simulink model "fullStateFeedback"  (R2019b)
settings: Solver=VariableStepAuto  StartTime=0.0  StopTime=3  RelTol=1e-3
values from neighbouring files (symbols this model uses):
  encGain = (2*pi)/4096    (= 0.00153398078789)    [DC_Motor_Analysis.m]    (also in Part2.m; Part3.m; lqrPoles.mat; robust.mat)
  feedForwardGain = 1/dcGain    [DC_Motor_Analysis.m]
  K = K_tilde(1:2)    [DC_Motor_Analysis.m]    (also in Part3.m = double(linsolve(meatMat, potatoesMat)))
settings Model: Creator=justinf  LastModifiedBy=justinf

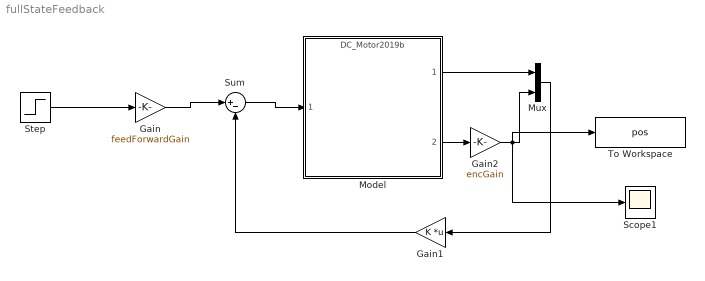
== system fullStateFeedback ==
  Gain : Gain  Gain=feedForwardGain
  Gain1 : Gain  Gain=K  Multiplication=Matrix(K*u)
  Gain2 : Gain  Gain=encGain
  Model : ModelReference  ModelNameDialog=DC_Motor2019b.slxp  ModelReferenceVersion=1.20  CopyOfModelProtected=on
  Mux : Mux  Inputs=2
  Scope1 : Scope
  Step : Step  Time=0  SampleTime=0
  Sum : Sum  Inputs=|+-
  To Workspace : ToWorkspace  VariableName=pos  SampleTime=-1
  wires:
  Sum/1 -> Model/1
  Step/1 -> Gain/1
  Gain1/1 -> Sum/2
  Model/1 -> Mux/1
  Mux/1 -> Gain1/1
  Gain/1 -> Sum/1
  Model/2 -> Gain2/1
  Gain2/1 -> Scope1/1, To Workspace/1, Mux/2
